simulink model "Bai_4_5"  (R2020b)
settings: Solver=VariableStepAuto  StartTime=0.0  StopTime=10.0  RelTol=1e-3
libraries: simulink x1
settings Model: Creator=John Andrew  LastModifiedBy=John Andrew

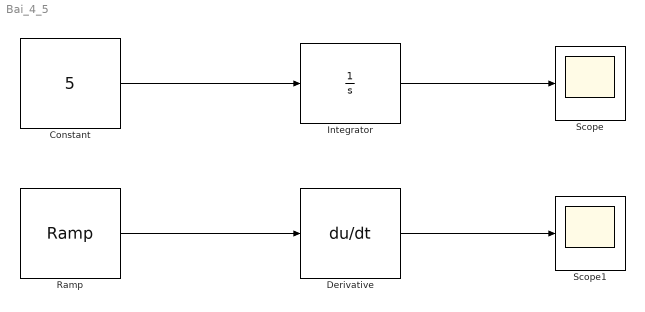
== system Bai_4_5 ==
  Constant : Constant  Value=5
  Derivative : Derivative
  Integrator : Integrator
  Ramp : simulink/Sources/Ramp  slope=1  start=0  InitialOutput=0
  Scope : Scope
  Scope1 : Scope
  wires:
  Constant/1 -> Integrator/1
  Ramp/1 -> Derivative/1
  Integrator/1 -> Scope/1
  Derivative/1 -> Scope1/1
